simulink model "IntelligentFan(1)"  (R2023b)
settings: Solver=ode23t  StartTime=0.0  StopTime=6  MaxStep=1e-5  RelTol=1e-3  EnableMultiTasking=on
libraries: fuzblock x1
settings Model: Creator=Rhoever
settings SolverCC: AlgebraicLoopSolver=TrustRegion
settings DataIOCC: LimitDataPoints=on  SaveFormat=Array  ReturnWorkspaceOutputs=off
settings OptimizationCC: LifeSpan=inf
settings DebuggingCC: SolverPrmCheckMsg=warning  UnconnectedInputMsg=warning  UnconnectedOutputMsg=warning  UnconnectedLineMsg=warning  SFUnexpectedBacktrackingDiag=warning  SFNoUnconditionalDefaultTransitionDiag=warning  SFExecutionAtInitializationDiag=none  ArithmeticOperatorsInVariantConditions=warning
settings HardwareCC: ProdBitPerPointer=32  ProdBitPerSizeT=32  ProdBitPerPtrDiffT=32  ProdLargestAtomicFloat=None  ProdIntDivRoundTo=Undefined  ProdEndianess=Unspecified  ProdWordSize=32  ProdHWDeviceType=32-bit Generic
settings ModelReferenceCC: EnableRefExpFcnMdlSchedulingChecks=on  PropagateSignalLabelsOutOfModel=off
settings SFSimCC: SimUseLocalCustomCode=off  CustomCodeUndefinedFunction=UseInterfaceOnly
settings RTWCC: RTWUseLocalCustomCode=off
settings CodeAppCC: StateflowObjectComments=on
settings GRTTargetCC: TargetLangStandard=C89/C90 (ANSI)
settings ConfigComp: CovMetricSettings=dw  CovSaveCumulativeToWorkspaceVar=on  CovSaveSingleToWorkspaceVar=on  CovExternalEMLEnable=off  CovSFcnEnable=off
settings SimscapeCC: SimscapeNormalizeSystem=off
settings ConfigurationSet: Description=SimMechanics 2G

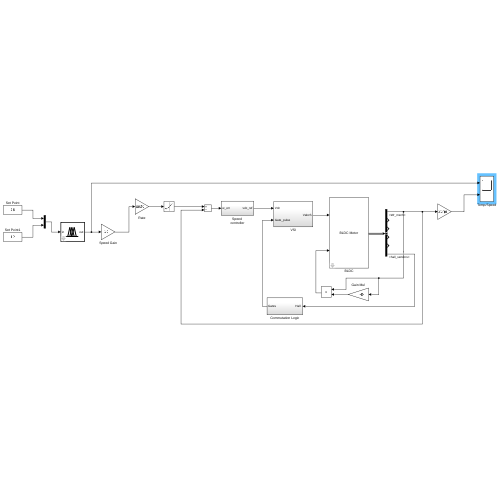
[thumbnail: Simulink's stored preview of the top-level diagram]
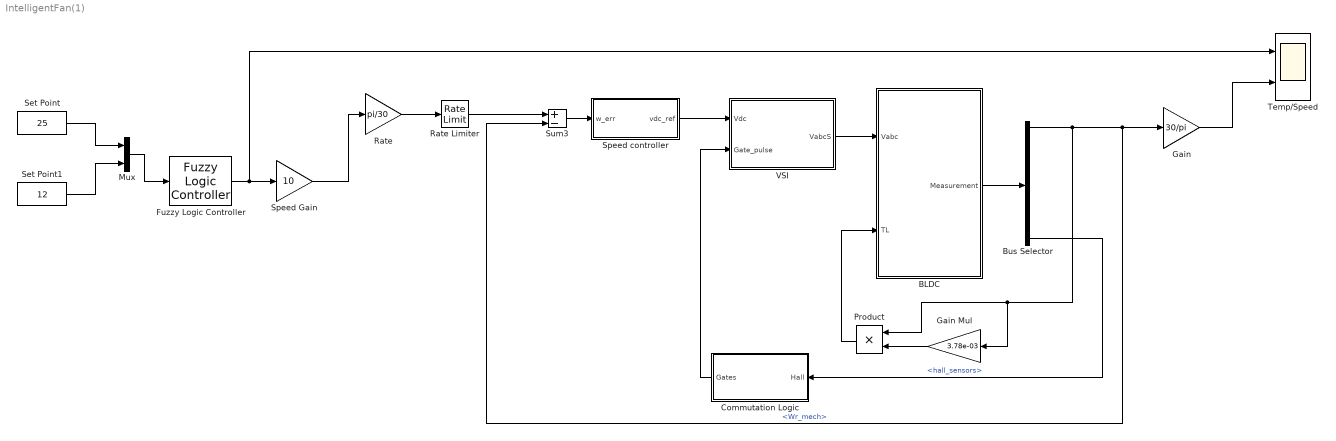
== system IntelligentFan(1) ==
  BLDC : Subsystem  mask(BLDC Motor :){Rs=1.43, Lls=9.4e-3, Phi_m=0.2158, J=5.5e-3, B=2e-3, P=4}
      mask prompts: Rs "Resistance - Rs [ohms]"; Lls "Inductance - Lls [H]"; Phi_m "Rotor Flux [wb]"; J "Rotor Inertia - J [kg-m^2]"; B "Friction Coefficient -B"; P "No of Poles"
      mask init:
      | Trap=0.5;
      mask Display: fprintf('BLDC Motor')
  Bus Selector : BusSelector  OutputSignals=Wr_mech,Te_vs_TL,Stator currents,trapezoidal rotor fluxes,eabc,hall_sensors
  Commutation Logic : Subsystem
  Fuzzy Logic Controller : fuzblock/Fuzzy Logic  Controller  FIS='myflcc.fis'  OutputSampleNumber=101  DataType=double  FuzzifiedInputs=off  RuleFiringStrengths=off  RuleOutputs=off  AggregatedOutputs=off  SimulateUsing=Interpreted execution  OutOfRangeInputValueMessage=warning  NoRuleFiredMessage=warning  EmptyOutputFuzzySetMessage=warning
  Gain : Gain  Gain=30/pi  SaturateOnIntegerOverflow=on  OutDataTypeStr=Inherit: Same as input  ParamDataTypeStr=Inherit: Same as input
  Gain Mul : Gain  Gain=3.78e-03
  Mux : Mux  Inputs=2
  Product : Product
  Rate : Gain  Gain=pi/30  SaturateOnIntegerOverflow=on  OutDataTypeStr=Inherit: Same as input  ParamDataTypeStr=Inherit: Same as input
  Rate Limiter : RateLimiter  RisingSlewLimit=75.4  FallingSlewLimit=-75.4  SampleTimeMode=inherited
  Set Point : Constant  Value=25
  Set Point1 : Constant  Value=12
  Speed controller : Subsystem
  Speed Gain : Gain  Gain=10  SaturateOnIntegerOverflow=on  OutDataTypeStr=Inherit: Same as input  ParamDataTypeStr=Inherit: Same as input
  Sum3 : Sum  Inputs=+-
  Temp/Speed : Scope  NumInputPorts=2
  VSI : Subsystem
  wires:
  Product/1 -> BLDC/2(TL)
  BLDC/1(Measurement) -> Bus Selector/1
  Bus Selector/6 -> Commutation Logic/1("Hall ")  "<hall_sensors>"
  VSI/1(VabcS) -> BLDC/1(Vabc)
  Commutation Logic/1(Gates) -> VSI/2(Gate_pulse)
  Sum3/1 -> Speed controller/1(w_err)
  Rate Limiter/1 -> Sum3/1
  Speed controller/1(vdc_ref) -> VSI/1(Vdc)
  Bus Selector/1 -> Gain Mul/1, Product/1, Gain/1, Sum3/2  "<Wr_mech>"
  Gain Mul/1 -> Product/2
  Rate/1 -> Rate Limiter/1
  Gain/1 -> Temp/Speed/2
  Speed Gain/1 -> Rate/1
  Fuzzy Logic Controller/1 -> Temp/Speed/1, Speed Gain/1
  Set Point/1 -> Mux/1
  Set Point1/1 -> Mux/2
  Mux/1 -> Fuzzy Logic Controller/1

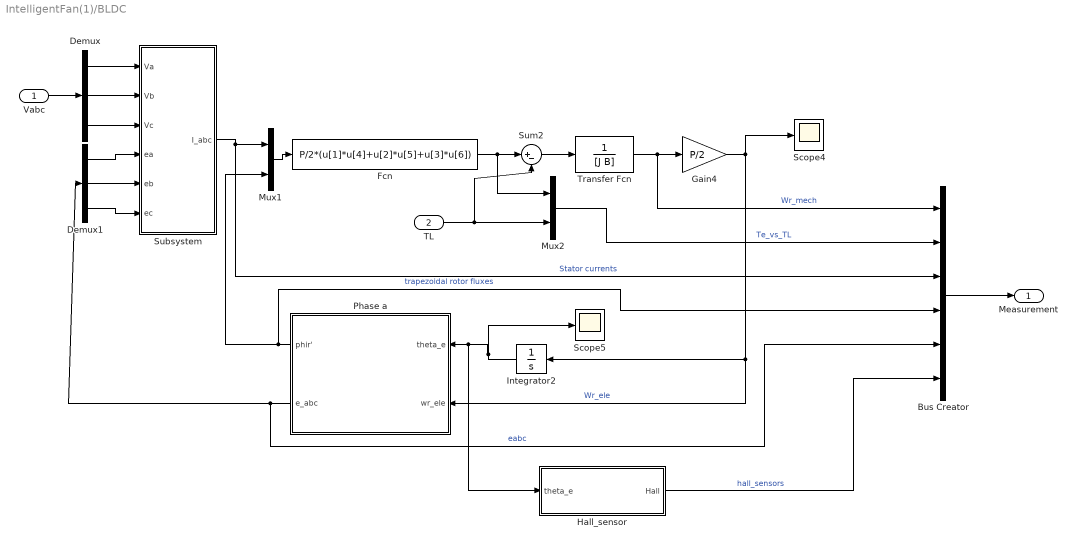
== system IntelligentFan(1)/BLDC ==
  Vabc : Inport
  TL : Inport  Port=2
  Bus Creator : BusCreator  Inputs=6
  Demux : Demux  Outputs=3
  Demux1 : Demux  Outputs=3
  Fcn : Fcn  Expr=P/2*(u[1]*u[4]+u[2]*u[5]+u[3]*u[6])
  Gain4 : Gain  Gain=P/2
  Hall_sensor : Subsystem
  Integrator2 : Integrator
  Mux1 : Mux  Inputs=2
  Mux2 : Mux  Inputs=2
  Phase a : Subsystem
  Scope4 : Scope
  Scope5 : Scope
  Subsystem : Subsystem
  Sum2 : Sum  Inputs=|+-
  Transfer Fcn : TransferFcn  Denominator=[J B]
  Measurement : Outport
  wires:
  Demux/3 -> Subsystem/3(Vc)
  Demux/1 -> Subsystem/1(Va)
  Demux/2 -> Subsystem/2(Vb)
  Sum2/1 -> Transfer Fcn/1
  Vabc/1 -> Demux/1
  Mux1/1 -> Fcn/1
  Demux1/3 -> Subsystem/6(ec)
  Demux1/2 -> Subsystem/5(eb)
  Demux1/1 -> Subsystem/4(ea)
  Integrator2/1 -> Hall_sensor/1(theta_e), Phase a/1(theta_e), Scope5/1
  Bus Creator/1 -> Measurement/1
  Transfer Fcn/1 -> Gain4/1, Bus Creator/1  "Wr_mech"
  TL/1 -> Sum2/2, Mux2/2
  Phase a/2(e_abc) -> Bus Creator/5, Demux1/1  "eabc"
  Gain4/1 -> Scope4/1, Phase a/2(wr_ele), Integrator2/1  "Wr_ele"
  Phase a/1(phir') -> Mux1/2, Bus Creator/4  "trapezoidal rotor fluxes"
  Subsystem/1(I_abc) -> Bus Creator/3, Mux1/1  "Stator currents"
  Fcn/1 -> Mux2/1, Sum2/1
  Hall_sensor/1(Hall) -> Bus Creator/6  "hall_sensors"
  Mux2/1 -> Bus Creator/2  "Te_vs_TL"

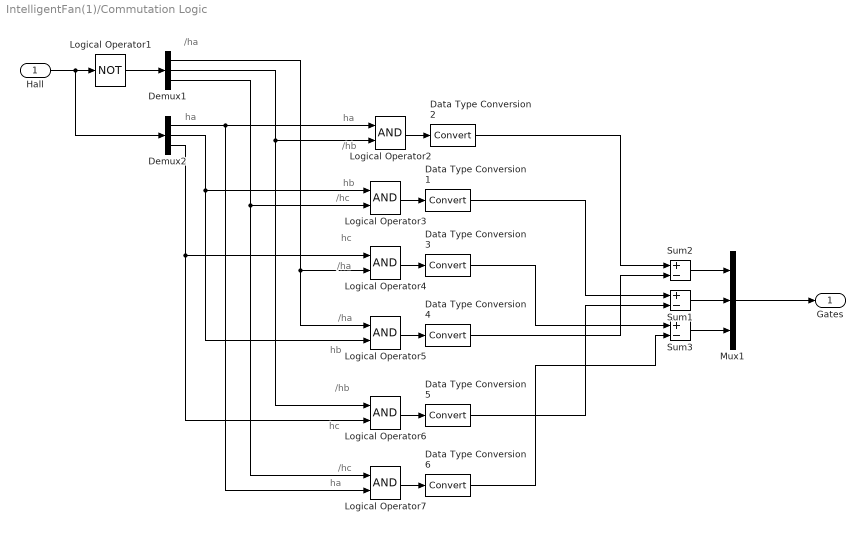
== system IntelligentFan(1)/Commutation Logic ==
  note: ha
  note: /hc
  note: hc
  note: /hb
  note: hb
  note: /ha
  note: /ha
  note: hc
  note: /hc
  note: hb
  note: /hb
  note: ha
  note: ha
  note: /ha
  "Hall " : Inport
  Data Type Conversion{1..6} (6 alike) : DataTypeConversion  SaturateOnIntegerOverflow=off  RndMeth=Floor
  Demux1 : Demux  Outputs=3
  Demux2 : Demux  Outputs=3
  Logical Operator1 : Logic  Operator=NOT  AllPortsSameDT=off  OutDataTypeStr=boolean
  Logical Operator{2..7} (6 alike) : Logic  AllPortsSameDT=off  OutDataTypeStr=boolean
  Mux1 : Mux  Inputs=3
  Sum1 : Sum  Inputs=+-  OutDataTypeStr=double
  Sum2 : Sum  Inputs=+-  OutDataTypeStr=double
  Sum3 : Sum  Inputs=+-  OutDataTypeStr=double
  Gates : Outport
  wires:
  Demux2/3 -> Logical Operator6/2, Logical Operator4/1
  Sum2/1 -> Mux1/1
  Mux1/1 -> Gates/1
  Logical Operator1/1 -> Demux1/1
  Logical Operator7/1 -> Data Type Conversion6/1
  Sum3/1 -> Mux1/3
  Logical Operator4/1 -> Data Type Conversion3/1
  Data Type Conversion4/1 -> Sum2/2
  Data Type Conversion5/1 -> Sum1/2
  Demux1/1 -> Logical Operator5/1, Logical Operator4/2
  Data Type Conversion3/1 -> Sum3/1
  Data Type Conversion6/1 -> Sum3/2
  Logical Operator5/1 -> Data Type Conversion4/1
  Data Type Conversion2/1 -> Sum2/1
  Logical Operator6/1 -> Data Type Conversion5/1
  Demux1/2 -> Logical Operator6/1, Logical Operator2/2
  Logical Operator2/1 -> Data Type Conversion2/1
  Logical Operator3/1 -> Data Type Conversion1/1
  "Hall "/1 -> Demux2/1, Logical Operator1/1
  Data Type Conversion1/1 -> Sum1/1
  Sum1/1 -> Mux1/2
  Demux2/2 -> Logical Operator5/2, Logical Operator3/1
  Demux1/3 -> Logical Operator7/1, Logical Operator3/2
  Demux2/1 -> Logical Operator7/2, Logical Operator2/1

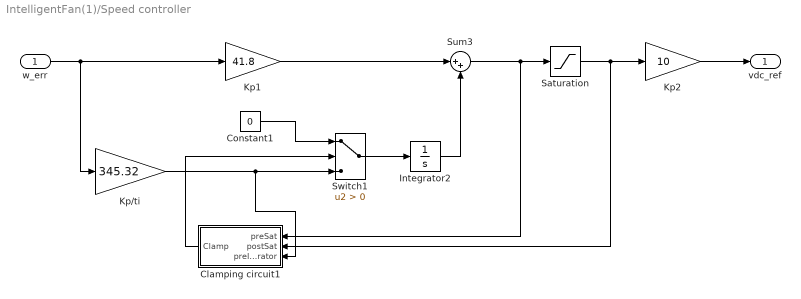
== system IntelligentFan(1)/Speed controller ==
  w_err : Inport
  Clamping circuit1 : Subsystem
  Constant1 : Constant  DisableCoverage=on  Value=0  OutDataTypeStr=Inherit: Inherit via back propagation  PreserveConstantTs=on
  Integrator2 : Integrator
  Kp/ti : Gain  Gain=345.32
  Kp1 : Gain  Gain=41.8
  Kp2 : Gain  Gain=10
  Saturation : Saturate  UpperLimit=15  LowerLimit=-15
  Sum3 : Sum  Inputs=|++
  Switch1 : Switch  DisableCoverage=on  Criteria=u2 > Threshold  SaturateOnIntegerOverflow=off
  vdc_ref : Outport
  wires:
  Kp1/1 -> Sum3/1
  Sum3/1 -> Saturation/1, Clamping circuit1/1(preSat)
  Saturation/1 -> Kp2/1, Clamping circuit1/2(postSat)
  w_err/1 -> Kp/ti/1, Kp1/1
  Kp2/1 -> vdc_ref/1
  Integrator2/1 -> Sum3/2
  Kp/ti/1 -> Switch1/3, Clamping circuit1/3(preIntegrator)
  Clamping circuit1/1(Clamp) -> Switch1/2
  Switch1/1 -> Integrator2/1
  Constant1/1 -> Switch1/1

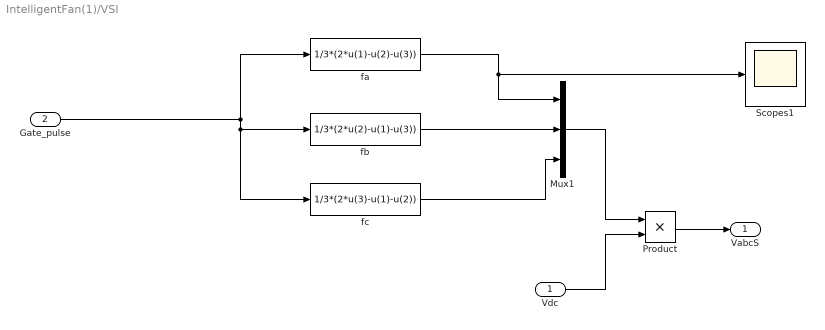
== system IntelligentFan(1)/VSI ==
  Vdc : Inport
  Gate_pulse : Inport  Port=2
  Mux1 : Mux  Inputs=3
  Product : Product
  Scopes1 : Scope
  fa : Fcn  Expr=1/3*(2*u(1)-u(2)-u(3))
  fb : Fcn  Expr=1/3*(2*u(2)-u(1)-u(3))
  fc : Fcn  Expr=1/3*(2*u(3)-u(1)-u(2))
  VabcS : Outport
  wires:
  Gate_pulse/1 -> fa/1, fb/1, fc/1
  fb/1 -> Mux1/2
  fc/1 -> Mux1/3
  fa/1 -> Scopes1/1, Mux1/1
  Mux1/1 -> Product/1
  Product/1 -> VabcS/1
  Vdc/1 -> Product/2

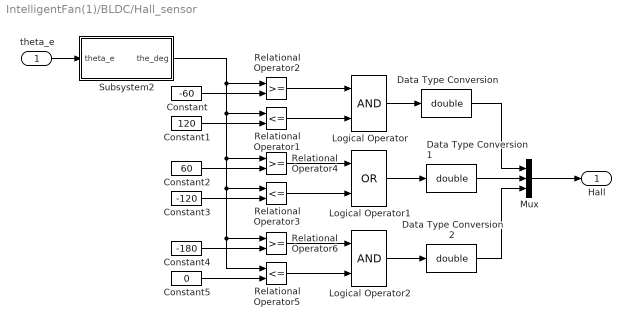
== system IntelligentFan(1)/BLDC/Hall_sensor ==
  theta_e : Inport
  Constant : Constant  Value=-60
  Constant1 : Constant  Value=120
  Constant2 : Constant  Value=60
  Constant3 : Constant  Value=-120
  Constant4 : Constant  Value=-180
  Constant5 : Constant  Value=0
  Data Type Conversion : DataTypeConversion  OutDataTypeStr=double
  Data Type Conversion1 : DataTypeConversion  OutDataTypeStr=double
  Data Type Conversion2 : DataTypeConversion  OutDataTypeStr=double
  Logical Operator : Logic  AllPortsSameDT=off  OutDataTypeStr=boolean
  Logical Operator1 : Logic  Operator=OR  AllPortsSameDT=off  OutDataTypeStr=boolean
  Logical Operator2 : Logic  AllPortsSameDT=off  OutDataTypeStr=boolean
  Mux : Mux  Inputs=3
  Relational Operator1 : RelationalOperator  Operator=<=
  Relational Operator2 : RelationalOperator
  Relational Operator3 : RelationalOperator  Operator=<=
  Relational Operator4 : RelationalOperator
  Relational Operator5 : RelationalOperator  Operator=<=
  Relational Operator6 : RelationalOperator
  Subsystem2 : Subsystem
  Hall : Outport
  wires:
  Constant3/1 -> Relational Operator3/2
  Data Type Conversion2/1 -> Mux/3
  Data Type Conversion1/1 -> Mux/2
  Data Type Conversion/1 -> Mux/1
  Relational Operator5/1 -> Logical Operator2/2
  Logical Operator2/1 -> Data Type Conversion2/1
  Relational Operator6/1 -> Logical Operator2/1
  Constant4/1 -> Relational Operator6/2
  Constant5/1 -> Relational Operator5/2
  Relational Operator3/1 -> Logical Operator1/2
  Logical Operator1/1 -> Data Type Conversion1/1
  Logical Operator/1 -> Data Type Conversion/1
  Mux/1 -> Hall/1
  Relational Operator2/1 -> Logical Operator/1
  Relational Operator1/1 -> Logical Operator/2
  Subsystem2/1(the_deg) -> Relational Operator4/1, Relational Operator3/1, Relational Operator5/1, Relational Operator6/1, Relational Operator1/1, Relational Operator2/1
  Constant/1 -> Relational Operator2/2
  Relational Operator4/1 -> Logical Operator1/1
  Constant1/1 -> Relational Operator1/2
  Constant2/1 -> Relational Operator4/2
  theta_e/1 -> Subsystem2/1(theta_e)

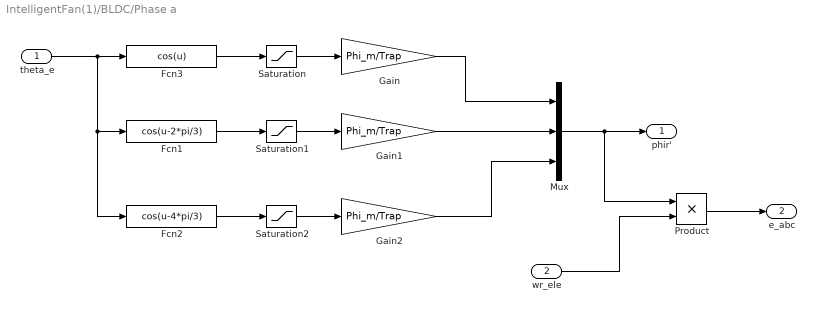
== system IntelligentFan(1)/BLDC/Phase a ==
  theta_e : Inport
  wr_ele : Inport  Port=2
  Fcn1 : Fcn  Expr=cos(u-2*pi/3)
  Fcn2 : Fcn  Expr=cos(u-4*pi/3)
  Fcn3 : Fcn  Expr=cos(u)
  Gain : Gain  Gain=Phi_m/Trap
  Gain1 : Gain  Gain=Phi_m/Trap
  Gain2 : Gain  Gain=Phi_m/Trap
  Mux : Mux  Inputs=3
  Product : Product
  Saturation : Saturate  UpperLimit=Trap  LowerLimit=-Trap
  Saturation1 : Saturate  UpperLimit=Trap  LowerLimit=-Trap
  Saturation2 : Saturate  UpperLimit=Trap  LowerLimit=-Trap
  phir' : Outport
  e_abc : Outport  Port=2
  wires:
  Fcn3/1 -> Saturation/1
  theta_e/1 -> Fcn2/1, Fcn1/1, Fcn3/1
  Fcn2/1 -> Saturation2/1
  Fcn1/1 -> Saturation1/1
  Gain/1 -> Mux/1
  Gain1/1 -> Mux/2
  Gain2/1 -> Mux/3
  Mux/1 -> phir'/1, Product/1
  wr_ele/1 -> Product/2
  Product/1 -> e_abc/1
  Saturation/1 -> Gain/1
  Saturation1/1 -> Gain1/1
  Saturation2/1 -> Gain2/1

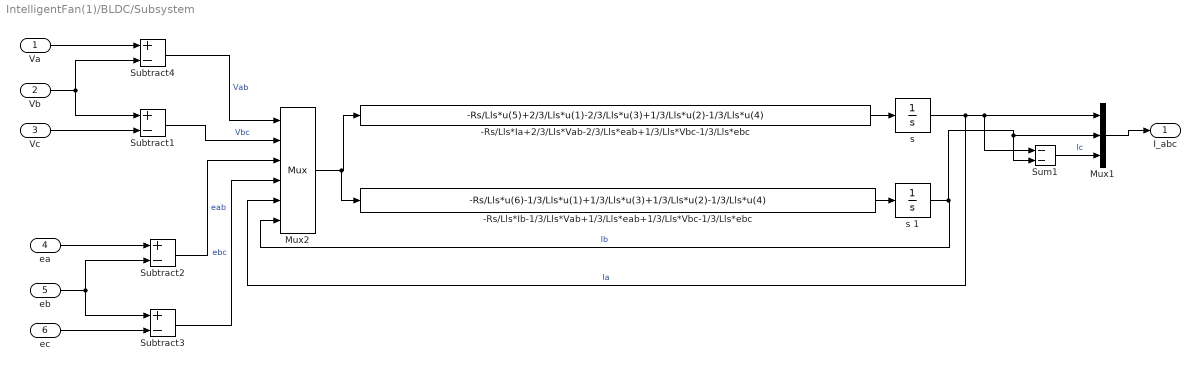
== system IntelligentFan(1)/BLDC/Subsystem ==
  Va : Inport
  Vb : Inport  Port=2
  Vc : Inport  Port=3
  ea : Inport  Port=4
  eb : Inport  Port=5
  ec : Inport  Port=6
  -Rs/Lls*Ia+2/3/Lls*Vab-2/3/Lls*eab+1/3/Lls*Vbc-1/3/Lls*ebc : Fcn  Expr=-Rs/Lls*u(5)+2/3/Lls*u(1)-2/3/Lls*u(3)+1/3/Lls*u(2)-1/3/Lls*u(4)
  -Rs/Lls*Ib-1/3/Lls*Vab+1/3/Lls*eab+1/3/Lls*Vbc-1/3/Lls*ebc : Fcn  Expr=-Rs/Lls*u(6)-1/3/Lls*u(1)+1/3/Lls*u(3)+1/3/Lls*u(2)-1/3/Lls*u(4)
  Mux1 : Mux  Inputs=3
  Mux2 : Mux  Inputs=6
      settings: DisplayOption=signals
  Subtract{1..4} (4 alike) : Sum  Inputs=+-
  Sum1 : Sum  Inputs=--  SaturateOnIntegerOverflow=on
  "s " : Integrator
  s 1 : Integrator
  I_abc : Outport
  wires:
  Va/1 -> Subtract4/1
  Vb/1 -> Subtract4/2, Subtract1/1
  Vc/1 -> Subtract1/2
  eb/1 -> Subtract2/2, Subtract3/1
  ea/1 -> Subtract2/1
  ec/1 -> Subtract3/2
  -Rs/Lls*Ia+2/3/Lls*Vab-2/3/Lls*eab+1/3/Lls*Vbc-1/3/Lls*ebc/1 -> "s "/1
  Subtract3/1 -> Mux2/4  "ebc"
  -Rs/Lls*Ib-1/3/Lls*Vab+1/3/Lls*eab+1/3/Lls*Vbc-1/3/Lls*ebc/1 -> s 1/1
  Subtract4/1 -> Mux2/1  "Vab"
  Subtract1/1 -> Mux2/2  "Vbc"
  Subtract2/1 -> Mux2/3  "eab"
  Mux2/1 -> -Rs/Lls*Ib-1/3/Lls*Vab+1/3/Lls*eab+1/3/Lls*Vbc-1/3/Lls*ebc/1, -Rs/Lls*Ia+2/3/Lls*Vab-2/3/Lls*eab+1/3/Lls*Vbc-1/3/Lls*ebc/1
  s 1/1 -> Sum1/2, Mux1/2, Mux2/6  "Ib"
  "s "/1 -> Sum1/1, Mux1/1, Mux2/5  "Ia"
  Sum1/1 -> Mux1/3  "Ic"
  Mux1/1 -> I_abc/1

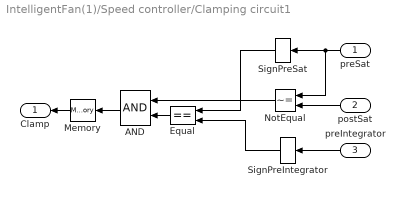
== system IntelligentFan(1)/Speed controller/Clamping circuit1 ==
  preSat : Inport
  postSat : Inport  Port=2
  preIntegrator : Inport  Port=3
  AND : Logic  DisableCoverage=on  OutDataTypeStr=boolean
  Equal : RelationalOperator  DisableCoverage=on  Operator===  OutDataTypeStr=boolean
  Memory : Memory
  NotEqual : RelationalOperator  DisableCoverage=on  Operator=~=  OutDataTypeStr=boolean
  SignPreIntegrator : Signum  DisableCoverage=on
  SignPreSat : Signum  DisableCoverage=on
  Clamp : Outport
  wires:
  Memory/1 -> Clamp/1
  AND/1 -> Memory/1
  Equal/1 -> AND/2
  SignPreIntegrator/1 -> Equal/2
  NotEqual/1 -> AND/1
  SignPreSat/1 -> Equal/1
  preIntegrator/1 -> SignPreIntegrator/1
  postSat/1 -> NotEqual/2
  preSat/1 -> NotEqual/1, SignPreSat/1

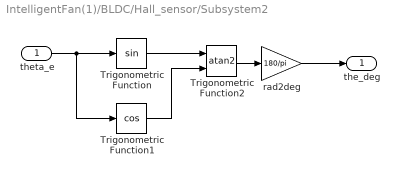
== system IntelligentFan(1)/BLDC/Hall_sensor/Subsystem2 ==
  theta_e : Inport
  Trigonometric Function : Trigonometry
  Trigonometric Function1 : Trigonometry  Operator=cos
  Trigonometric Function2 : Trigonometry  Operator=atan2
  rad2deg : Gain  Gain=180/pi  SaturateOnIntegerOverflow=on  OutDataTypeStr=Inherit: Same as input  ParamDataTypeStr=Inherit: Same as input
  the_deg : Outport
  wires:
  Trigonometric Function2/1 -> rad2deg/1
  Trigonometric Function/1 -> Trigonometric Function2/1
  Trigonometric Function1/1 -> Trigonometric Function2/2
  theta_e/1 -> Trigonometric Function1/1, Trigonometric Function/1
  rad2deg/1 -> the_deg/1
